simulink model "atrias_HW_boom_nmSt_kinSw"  (R2015a)
settings: Solver=ode4  StartTime=0.0  StopTime=inf  FixedStep=sample_time  RelTol=1e-3
values from neighbouring files (symbols this model uses):
  control_start_time = 15    [setParams.m]
  flag_CtrlMode = 0    [setParams.m]
  kinSw_t_start = 0.5    [setParams.m]
  poser_LLegAlp = (initial_l_leg_angle -pi/2)*180/pi    (= 105)    [setParams.m]
  poser_LLegLen = initial_l_leg_length    (= 0.8)    [setParams.m]
  poser_RLegAlp = (initial_r_leg_angle -pi/2)*180/pi    (= 75)    [setParams.m]
  poser_RLegLen = initial_r_leg_length    (= 0.8)    [setParams.m]
  tune_kinSw_alpha_start = kinSw_alpha_start*180/pi    (= 130)    [setParams.m]
  tune_kinSw_alpha_tgt = kinSw_alpha_tgt*180/pi    (= 80)    [setParams.m]
  tune_kinSw_len_min = kinSw_len_min    (= 0.7)    [setParams.m]
  tune_kinSw_len_tgt = kinSw_len_tgt    (= 0.9)    [setParams.m]
  tune_kinSw_min_t_del = kinSw_min_t_del    (= 0.425)    [setParams.m]
  tune_kinSw_t_del = kinSw_t_del    (= 0.5)    [setParams.m]
  tune_M1_G = St_FGain_VAS*FmaxVAS    [setParams.m]
  tune_M3_0 = CtrlPar_theta0*180/pi    [setParams.m]
  tune_M3_D = St_GainDTh_HFL    [setParams.m]
  tune_M3_P = St_GainTh_HFL    [setParams.m]
undefined symbols (not defined in the file or in its folder): A1_notch_f1, A2_notch_f1, A_kalman_fourbar_gear, A_lpf_dtau, B1_lpf_dtau, B1_notch_f1, B2_lpf_dtau, B2_notch_f1, B_kalman_fourbar_gear, boom_mount_angle, boom_mount_to_center_diagonal, c_jointstop, C_kalman_fourbar_gear, contactThr, d_vertical_com, delta_phi_max, delta_phi_max_buffer, delta_phi_max_dropoff, delta_phi_min, Discrete, FmaxBFSH, FmaxGLU, FmaxHAM, FmaxHFL, FmaxRF, FmaxVAS, FPCtrlPar, g, gain_nodes_sea_torque, HIP_MTR_MAX_CONT_TORQUE, initial_dx_estimate, j_motor, k_leg_spring, K_notch_f1, k_sea, kalman_load_to_deflect_transmission, kd_lateral, kd_motor, kd_shin_max, kd_shin_min, kd_splay_max, kd_splay_min, kd_thigh_max, kd_thigh_min, kp_lateral, kp_motor, kp_sea_torque, kp_shin_max, kp_shin_min, kp_splay_max, kp_splay_min, kp_thigh_max, kp_thigh_min, l_boom, l_seg, l_v, lateral_motor_efficiency, lateral_offset, lateral_target_angle_right, lateral_transition_force ... (+124)
libraries: simulink_extras x44, simulink x9, ctrlSharedLib x4
(part 2 of 8)

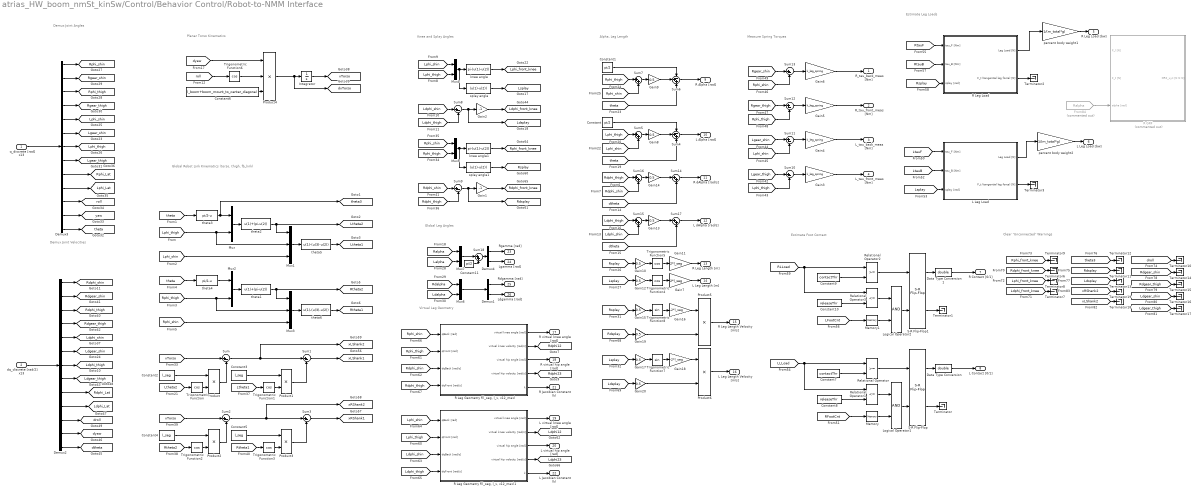
== system atrias_HW_boom_nmSt_kinSw/Control/Behavior Control/Robot-to-NMM Interface ==
  note: Global Robot Link Kinematics
      | (torso, thigh, fb_link)
  note: Planar Torso Kinematics
  note: Alpha, Leg Length
  note: Demux Joint
      | Angles
  note: Demux Joint
      | Velocities
  note: Knee and Splay Angles
  note: Virtual Leg Geometry
  note: Measure Spring Torques
  note: Estimate Leg Loads
  note: Estimate Foot Contact
  note: Clear "Unconnected" Warnings
  note: Global Leg Angles
  q_discrete [rad] x13 : Inport
  dq_discrete [rad/2] x13 : Inport  Port=2
  Constant : Constant  Value=pi/2
  Constant1 : Constant  Value=pi/2
  Constant10 : Constant  Value=releaseThr
  Constant11 : Constant  Value=pi/2
  Constant{2..5} (4 alike) : Constant  Value=l_seg
  Constant6 : Constant  Value=l_boom+boom_mount_to_center_diagonal
  Constant7 : Constant  Value=contactThr
  Constant8 : Constant  Value=releaseThr
  Constant9 : Constant  Value=contactThr
  Data Type Conversion : DataTypeConversion  OutDataTypeStr=double
  Data Type Conversion1 : DataTypeConversion  OutDataTypeStr=double
  Demux1 : Demux  Outputs=2
  Demux2 : Demux  Outputs=13
  Demux3 : Demux  Outputs=13
  Demux4 : Demux  Outputs=2
  From84 : From  Commented=on  GotoTag=Ralpha  TagVisibility=global
  Gain1 : Gain  Gain=-1
  Gain{8..10,12..15,17,19..20} (10 alike) : Gain  Gain=0.5
  Gain11 : Gain  Gain=2*l_seg
  Gain16 : Gain  Gain=-2*l_seg
  Gain18 : Gain  Gain=-2*l_seg
  Gain2 : Gain  Gain=-1
  Gain{3..6} (4 alike) : Gain  Gain=k_leg_spring
  Gain7 : Gain  Gain=2*l_seg
  Integrator : Integrator
  L Leg Load : Subsystem
  Logical Operator1 : Logic  AllPortsSameDT=off  OutDataTypeStr=boolean
  Logical Operator2 : Logic  AllPortsSameDT=off  OutDataTypeStr=boolean
  Memory : Memory
  Memory1 : Memory
  Mux{,2,4..7} (6 alike) : Mux  Inputs=2
  Mux1 : Mux  Inputs=3
  Mux3 : Mux  Inputs=3
  Product{,1..3,5..6} (6 alike) : Product
  Product4 : Product  Inputs=3
  R GRF : Subsystem  Commented=on
  "R Leg Geometry f(l_seg, l_v, v12_max)" : Subsystem
  "R Leg Geometry f(l_seg, l_v, v12_max)1" : Subsystem
  R Leg Load : Subsystem
  Relational Operator : RelationalOperator  OutDataTypeStr=boolean
  Relational Operator1 : RelationalOperator  Operator=<=  OutDataTypeStr=boolean
  Relational Operator2 : RelationalOperator  OutDataTypeStr=boolean
  Relational Operator3 : RelationalOperator  Operator=<=  OutDataTypeStr=boolean
  S-R Flip-Flop : simulink_extras/Flip Flops/S-R Flip-Flop  initial_condition=0
  S-R Flip-Flop1 : simulink_extras/Flip Flops/S-R Flip-Flop  initial_condition=0
  Sum{,1..3,8..13} (10 alike) : Sum  Inputs=|+-
  Sum{5,7,14..18} (7 alike) : Sum  Inputs=|++
  Sum4 : Sum  Inputs=-++
  Sum6 : Sum  Inputs=-++
  Terminator{,1..3,6..19} (18 alike) : Terminator
  Trigonometric Function{,1..6} (7 alike) : Trigonometry  Operator=cos
  Trigonometric Function7 : Trigonometry
  Trigonometric Function8 : Trigonometry
  knee angle : Fcn  Expr=pi-(u(1)-u(2))
  knee angle1 : Fcn  Expr=pi-(u(1)-u(2))
  percent body weight1 : Gain  Gain=1/(m_total*g)
  percent body weight2 : Gain  Gain=1/(m_total*g)
  splay angle : Fcn  Expr=(u(1)-u(2))
  splay angle1 : Fcn  Expr=(u(1)-u(2))
  theta1 : Fcn  Expr=u(1)+(pi-u(2))
  theta2 : Fcn  Expr=u(1)+(pi-u(2))
  theta3 : Fcn  Expr=pi/2-u
  theta4 : Fcn  Expr=pi/2-u
  theta5 : Fcn  Expr=u(1)-(u(3)-u(2))
  theta6 : Fcn  Expr=u(1)-(u(3)-u(2))
  R_tau_back_meas [Nm] : Outport
  R_tau_front_meas [Nm] : Outport  Port=2
  L_tau_back_meas [Nm] : Outport  Port=3
  L_tau_front_meas [Nm] : Outport  Port=4
  R Leg Load [bw] : Outport  Port=5
  L Leg Load [bw] : Outport  Port=6
  R Contact [0/1] : Outport  Port=7
  L Contact [0/1] : Outport  Port=8
  R Alpha [rad] : Outport  Port=9
  L Alpha [rad] : Outport  Port=10
  R dAlpha [rad/s] : Outport  Port=11
  L dAlpha [rad/s] : Outport  Port=12
  R Leg Length [m] : Outport  Port=13
  L Leg Length [m] : Outport  Port=14
  R Leg Length Velocity [m/s] : Outport  Port=15
  L Leg Length Velocity [m/s] : Outport  Port=16
  R virtual knee angle [rad] : Outport  Port=17
  R virtual hip angle [rad] : Outport  Port=18
  L virtual knee angle [rad] : Outport  Port=19
  L virtual hip angle [rad] : Outport  Port=20
  R Jacobian Constant (k) : Outport  Port=21
  L Jacobian Constant (k) : Outport  Port=22
  Rgamma [rad] : Outport  Port=23
  Lgamma [rad] : Outport  Port=24
  Rdgamma [rad] : Outport  Port=25
  Ldgamma [rad] : Outport  Port=26
  tag scope: Ldgear_shin=global, Ldgear_thigh=global, Ldphi12=global, Ldphi23=global, Ldphi_Lat=global, Ldphi_front_knee=global, Ldphi_shin=global, Ldphi_thigh=global, Ldsplay=global, Lgear_shin=global, Lgear_thigh=global, Lphi_Lat=global, Lphi_front_knee=global, Lphi_shin=global, Lphi_thigh=global, Lsplay=global, Ltheta1=global, Ltheta2=global, Rdgear_shin=global, Rdgear_thigh=global, Rdphi12=global, Rdphi23=global, Rdphi_Lat=global, Rdphi_front_knee=global, Rdphi_shin=global, Rdphi_thigh=global, Rdsplay=global, Rgear_shin=global, Rgear_thigh=global, Rphi_Lat=global, Rphi_front_knee=global, Rphi_shin=global, Rphi_thigh=global, Rsplay=global, Rtheta1=global, Rtheta2=global, droll=global, dtheta=global, dxTorso=global, dyaw=global, roll=global, theta3=global, theta=global, xLShank1=global, xLShank2=global, xRShank1=global, xRShank2=global, xTorso=global, yaw=global
  wires:
  Sum3/1 -> [xRShank1]
  Sum2/1 -> [xRShank2], Sum3/1
  Product3/1 -> Sum3/2
  Trigonometric Function3/1 -> Product3/2
  Constant2/1 -> Product/1
  Trigonometric Function/1 -> Product/2
  Sum1/1 -> [xLShank1]
  Constant3/1 -> Product1/1
  Trigonometric Function2/1 -> Product2/2
  Product1/1 -> Sum1/2
  [Rtheta2] -> Trigonometric Function2/1
  Sum/1 -> [xLShank2], Sum1/1
  [Ltheta1] -> Trigonometric Function1/1
  Product/1 -> Sum/2
  Product2/1 -> Sum2/2
  [xTorso] -> Sum2/1
  [Rtheta1] -> Trigonometric Function3/1
  Constant4/1 -> Product2/1
  Constant5/1 -> Product3/1
  [xTorso] -> Sum/1
  [Ltheta2] -> Trigonometric Function/1
  Product4/1 -> [dxTorso], Integrator/1
  Trigonometric Function1/1 -> Product1/2
  Integrator/1 -> [xTorso]
  [dyaw] -> Product4/1
  [theta] -> theta3/1
  [Lphi_thigh] -> Mux1/2, Mux/2
  theta3/1 -> Mux/1, [theta3]
  Mux/1 -> theta2/1
  theta2/1 -> Mux1/1, [Ltheta2]
  Mux1/1 -> theta5/1
  [Lphi_shin] -> Mux1/3
  [theta] -> theta4/1
  [Rphi_thigh] -> Mux3/2, Mux2/2
  theta4/1 -> Mux2/1
  Mux2/1 -> theta1/1
  theta1/1 -> Mux3/1, [Rtheta2]
  Mux3/1 -> theta6/1
  [Rphi_shin] -> Mux3/3
  theta5/1 -> [Ltheta1]
  theta6/1 -> [Rtheta1]
  [theta] -> Sum4/3
  Constant/1 -> Sum4/1
  [Lphi_thigh] -> Sum5/1
  [Lphi_shin] -> Sum5/2
  Sum5/1 -> Gain8/1
  Gain8/1 -> Sum4/2
  Sum4/1 -> L Alpha [rad]/1
  [theta] -> Sum6/3
  Constant1/1 -> Sum6/1
  [Rphi_thigh] -> Sum7/1
  [Rphi_shin] -> Sum7/2
  Sum7/1 -> Gain9/1
  Gain9/1 -> Sum6/2
  Sum6/1 -> R Alpha [rad]/1
  Gain12/1 -> Trigonometric Function4/1
  Gain10/1 -> Trigonometric Function5/1
  Trigonometric Function4/1 -> Gain7/1
  Trigonometric Function5/1 -> Gain11/1
  Demux3/1 -> [Rphi_shin]
  Demux3/2 -> [Rgear_shin]
  Demux3/3 -> [Rphi_thigh]
  Demux3/4 -> [Rgear_thigh]
  Demux3/5 -> [Lphi_shin]
  Demux3/6 -> [Lgear_shin]
  Demux3/7 -> [Lphi_thigh]
  Demux3/8 -> [Lgear_thigh]
  Demux3/9 -> [Rphi_Lat]
  Demux3/10 -> [Lphi_Lat]
  Demux3/11 -> [roll]
  Demux3/12 -> [yaw]
  Demux3/13 -> [theta]
  Demux2/13 -> [dtheta]
  Demux2/8 -> [Ldgear_thigh]
  Demux2/10 -> [Ldphi_Lat]
  Demux2/6 -> [Ldgear_shin]
  Demux2/9 -> [Rdphi_Lat]
  Demux2/11 -> [droll]
  Demux2/12 -> [dyaw]
  Demux2/4 -> [Rdgear_thigh]
  Demux2/5 -> [Ldphi_shin]
  Demux2/7 -> [Ldphi_thigh]
  Demux2/1 -> [Rdphi_shin]
  Demux2/3 -> [Rdphi_thigh]
  Demux2/2 -> [Rdgear_shin]
  q_discrete [rad] x13/1 -> Demux3/1
  dq_discrete [rad/2] x13/1 -> Demux2/1
  Mux4/1 -> splay angle/1, knee angle/1
  [Lphi_thigh] -> Mux4/2
  [Lphi_shin] -> Mux4/1
  knee angle/1 -> [Lphi_front_knee]
  [Ldphi_thigh] -> Sum8/2
  [Ldphi_shin] -> Sum8/1
  Sum8/1 -> [Ldsplay], Gain2/1
  Gain2/1 -> [Ldphi_front_knee]
  splay angle/1 -> [Lsplay]
  Trigonometric Function6/1 -> Product4/2
  [roll] -> Trigonometric Function6/1
  Constant6/1 -> Product4/3
  Mux5/1 -> splay angle1/1, knee angle1/1
  [Rphi_thigh] -> Mux5/2
  [Rphi_shin] -> Mux5/1
  knee angle1/1 -> [Rphi_front_knee]
  [Rdphi_thigh] -> Sum9/2
  [Rdphi_shin] -> Sum9/1
  Sum9/1 -> [Rdsplay], Gain1/1
  Gain1/1 -> [Rdphi_front_knee]
  splay angle1/1 -> [Rsplay]
  [Lgear_shin] -> Sum11/1
  Sum11/1 -> Gain4/1
  [Lphi_shin] -> Sum11/2
  Gain4/1 -> L_tau_back_meas [Nm]/1
  [Lgear_thigh] -> Sum10/1
  Sum10/1 -> Gain3/1
  [Lphi_thigh] -> Sum10/2
  Gain3/1 -> L_tau_front_meas [Nm]/1
  [Rgear_shin] -> Sum13/1
  Sum13/1 -> Gain6/1
  [Rphi_shin] -> Sum13/2
  Gain6/1 -> R_tau_back_meas [Nm]/1
  [Rgear_thigh] -> Sum12/1
  Sum12/1 -> Gain5/1
  [Rphi_thigh] -> Sum12/2
  Gain5/1 -> R_tau_front_meas [Nm]/1
  [Lsplay] -> L Leg Load/3(splay [rad])
  L Leg Load/1(Leg Load [N]) -> percent body weight2/1
  [LtauF] -> L Leg Load/1(tau_F [Nm])
  [LtauB] -> L Leg Load/2(tau_B [Nm])
  percent body weight2/1 -> L Leg Load [bw]/1
  Relational Operator/1 -> S-R Flip-Flop/1
  Constant7/1 -> Relational Operator/2
  S-R Flip-Flop/2 -> Terminator/1
  Logical Operator1/1 -> S-R Flip-Flop/2
  [RFootCnt] -> Memory/1
  Constant8/1 -> Relational Operator1/2
  Relational Operator1/1 -> Logical Operator1/1
  Memory/1 -> Logical Operator1/2
  Data Type Conversion/1 -> L Contact [0/1]/1
  S-R Flip-Flop/1 -> Data Type Conversion/1
  [LLLoad] -> Relational Operator/1, Relational Operator1/1
  [Rsplay] -> R Leg Load/3(splay [rad])
  R Leg Load/1(Leg Load [N]) -> percent body weight1/1
  [RtauF] -> R Leg Load/1(tau_F [Nm])
  [RtauB] -> R Leg Load/2(tau_B [Nm])
  percent body weight1/1 -> R Leg Load [bw]/1
  Relational Operator2/1 -> S-R Flip-Flop1/1
  Constant9/1 -> Relational Operator2/2
  S-R Flip-Flop1/2 -> Terminator1/1
  Logical Operator2/1 -> S-R Flip-Flop1/2
  [LFootCnt] -> Memory1/1
  Constant10/1 -> Relational Operator3/2
  Relational Operator3/1 -> Logical Operator2/1
  Memory1/1 -> Logical Operator2/2
  Data Type Conversion1/1 -> R Contact [0/1]/1
  S-R Flip-Flop1/1 -> Data Type Conversion1/1
  [RLLoad] -> Relational Operator3/1, Relational Operator2/1
  [Rsplay] -> Gain10/1
  [Lsplay] -> Gain12/1
  Gain11/1 -> R Leg Length [m]/1
  Gain7/1 -> L Leg Length [m]/1
  [Rphi_thigh] -> "R Leg Geometry f(l_seg, l_v, v12_max)"/2(qFront [rad])
  [Rphi_shin] -> "R Leg Geometry f(l_seg, l_v, v12_max)"/1(qBack [rad])
  [Rdphi_shin] -> "R Leg Geometry f(l_seg, l_v, v12_max)"/3(dqBack [rad/s])
  [Rdphi_thigh] -> "R Leg Geometry f(l_seg, l_v, v12_max)"/4(dqFront [rad/s])
  "R Leg Geometry f(l_seg, l_v, v12_max)"/4(virtual hip velocity [rad/s]) -> [Rdphi23]
  "R Leg Geometry f(l_seg, l_v, v12_max)"/2(virtual knee velocity [rad/s]) -> [Rdphi12]
  "R Leg Geometry f(l_seg, l_v, v12_max)"/5(k) -> R Jacobian Constant (k)/1
  [Lphi_thigh] -> "R Leg Geometry f(l_seg, l_v, v12_max)1"/2(qFront [rad])
  [Lphi_shin] -> "R Leg Geometry f(l_seg, l_v, v12_max)1"/1(qBack [rad])
  [Ldphi_shin] -> "R Leg Geometry f(l_seg, l_v, v12_max)1"/3(dqBack [rad/s])
  [Ldphi_thigh] -> "R Leg Geometry f(l_seg, l_v, v12_max)1"/4(dqFront [rad/s])
  "R Leg Geometry f(l_seg, l_v, v12_max)1"/5(k) -> L Jacobian Constant (k)/1
  "R Leg Geometry f(l_seg, l_v, v12_max)"/3(virtual hip angle [rad]) -> R virtual hip angle [rad]/1
  "R Leg Geometry f(l_seg, l_v, v12_max)"/1(virtual knee angle [rad]) -> R virtual knee angle [rad]/1
  "R Leg Geometry f(l_seg, l_v, v12_max)1"/1(virtual knee angle [rad]) -> L virtual knee angle [rad]/1
  "R Leg Geometry f(l_seg, l_v, v12_max)1"/3(virtual hip angle [rad]) -> L virtual hip angle [rad]/1
  "R Leg Geometry f(l_seg, l_v, v12_max)1"/2(virtual knee velocity [rad/s]) -> [Ldphi12]
  "R Leg Geometry f(l_seg, l_v, v12_max)1"/4(virtual hip velocity [rad/s]) -> [Ldphi23]
  [Rdphi_front_knee] -> Terminator6/1
  [Ldphi_front_knee] -> Terminator7/1
  [Lphi_front_knee] -> Terminator8/1
  [Rphi_front_knee] -> Terminator9/1
  [droll] -> Terminator10/1
  [Rdsplay] -> Terminator11/1
  [theta3] -> Terminator12/1
  [Ldsplay] -> Terminator13/1
  [Rdgear_shin] -> Terminator14/1
  [Rdgear_thigh] -> Terminator15/1
  [Ldgear_shin] -> Terminator16/1
  [Ldgear_thigh] -> Terminator17/1
  [xLShank2] -> Terminator18/1
  [xRShank2] -> Terminator19/1
  Sum17/1 -> L dAlpha [rad/s]/1
  Sum14/1 -> R dAlpha [rad/s]/1
  [Ldphi_thigh] -> Sum15/1
  [Ldphi_shin] -> Sum15/2
  Sum15/1 -> Gain13/1
  Gain13/1 -> Sum17/1
  [dtheta] -> Sum17/2
  [Rdphi_thigh] -> Sum16/1
  [Rdphi_shin] -> Sum16/2
  Sum16/1 -> Gain14/1
  Gain14/1 -> Sum14/1
  [dtheta] -> Sum14/2
  Constant11/1 -> Sum18/2
  [Ralpha] -> Mux7/1
  [Lalpha] -> Mux7/2
  Mux7/1 -> Sum18/1
  Sum18/1 -> Demux4/1
  Demux4/1 -> Rgamma [rad]/1
  Demux4/2 -> Lgamma [rad]/1
  [Rdalpha] -> Mux6/1
  [Ldalpha] -> Mux6/2
  Mux6/1 -> Demux1/1
  Demux1/1 -> Rdgamma [rad]/1
  Demux1/2 -> Ldgamma [rad]/1
  Gain15/1 -> Trigonometric Function8/1
  Trigonometric Function8/1 -> Gain16/1
  [Rsplay] -> Gain15/1
  Gain16/1 -> Product5/1
  [Rdsplay] -> Gain19/1
  Gain19/1 -> Product5/2
  Product5/1 -> R Leg Length Velocity [m/s]/1
  Gain17/1 -> Trigonometric Function7/1
  Trigonometric Function7/1 -> Gain18/1
  [Lsplay] -> Gain17/1
  Gain18/1 -> Product6/1
  [Ldsplay] -> Gain20/1
  Gain20/1 -> Product6/2
  Product6/1 -> L Leg Length Velocity [m/s]/1
  From84/1 -> R GRF/3(alpha [rad])
  R Leg Load/2(F_t (tangential leg force) [N]) -> Terminator2/1
  L Leg Load/2(F_t (tangential leg force) [N]) -> Terminator3/1

== system atrias_HW_boom_nmSt_kinSw/Control/Behavior Control/Subsystem ==
  R legL : Inport
  R phi : Inport  Port=2
  L legL : Inport  Port=3
  L phi : Inport  Port=4
  R BackGear : Inport  Port=5
  R Front Gear : Inport  Port=6
  L BackGear : Inport  Port=7
  L Front Gear : Inport  Port=8
  Lateral Torque Command [Nm Nm] : Inport  Port=9
  Avoid Hitting Mechanical Limits : MATLAB Function  TreatAsAtomicUnit=on
  Avoid Hitting Mechanical Limits1 : MATLAB Function  TreatAsAtomicUnit=on
  Back/Front Motor PD : Subsystem
  Back/Front Motor PD1 : Subsystem
  Constant1 : Constant
  Constant10 : Constant  Value=max_back_bar_angle
  Constant11 : Constant  Value=min_back_bar_angle
  Constant12 : Constant  Value=min_front_bar_angle
  Constant13 : Constant  Value=[0 0 0 0]  OutDataTypeStr=boolean
  Constant2 : Constant  Value=0
  Constant3 : Constant  Value=max_back_bar_angle
  Constant4 : Constant  Value=min_back_bar_angle
  Constant5 : Constant  Value=min_front_bar_angle
  Constant6 : Constant  Value=0
  Constant7 : Constant  Value=0
  Constant8 : Constant  Value=max_front_bar_angle
  Constant9 : Constant  Value=max_front_bar_angle
  Demux{1..4} (4 alike) : Demux  Outputs=2
  Mux{1..9,11} (10 alike) : Mux  Inputs=2
  Mux10 : Mux  Inputs=3
  Selector33 : Selector  InputPortWidth=6  Indices=[1 2 4 5]
  Selector8 : Selector  InputPortWidth=6  Indices=[1 2 5 3 4 6]
  Virtual Leg to Four Bar : MATLAB Function  TreatAsAtomicUnit=on
  Virtual Leg to Four Bar1 : MATLAB Function  TreatAsAtomicUnit=on
  dtau_des : Subsystem
  Motor Torque Command [Nm] x6 : Outport
  SEA Torque Velocity Command [Nm] x4 : Outport  Port=2
  Force / Position Control [1/0] x4 : Outport  Port=3
  wires:
  R phi/1 -> Virtual Leg to Four Bar/4(phi)
  Avoid Hitting Mechanical Limits/3(dback_cmd) -> Mux9/1
  Avoid Hitting Mechanical Limits/1(back_cmd) -> Mux5/1
  Mux6/1 -> Back/Front Motor PD/3(Desired Acceleration [rad/s^2] [back front])
  Constant9/1 -> Avoid Hitting Mechanical Limits/8(max_front_bar_angle)
  Constant11/1 -> Avoid Hitting Mechanical Limits/9(min_back_bar_angle)
  Constant1/1 -> Back/Front Motor PD/6(Right/Left Leg [1/0])
  R Front Gear/1 -> Demux1/1
  Constant12/1 -> Avoid Hitting Mechanical Limits/7(min_front_bar_angle)
  Demux1/1 -> Mux8/2
  Demux1/2 -> Mux11/2
  Virtual Leg to Four Bar/1(back) -> Avoid Hitting Mechanical Limits/1(back_desired)
  Virtual Leg to Four Bar/2(dback) -> Avoid Hitting Mechanical Limits/2(dback_desired)
  Demux2/1 -> Mux8/1
  Avoid Hitting Mechanical Limits/2(front_cmd) -> Mux5/2
  Virtual Leg to Four Bar/5(dfront) -> Avoid Hitting Mechanical Limits/5(dfront_desired)
  Demux2/2 -> Mux11/1
  R BackGear/1 -> Demux2/1
  Virtual Leg to Four Bar/4(front) -> Avoid Hitting Mechanical Limits/4(front_desired)
  Back/Front Motor PD/1(Commanded Torque [Nm] [back front]) -> [RCommandTorque_back_front]
  Virtual Leg to Four Bar/6(ddfront) -> Avoid Hitting Mechanical Limits/6(ddfront_desired)
  Mux11/1 -> Back/Front Motor PD/5(Measured Velocity [rad/s] [back front])
  Mux8/1 -> Back/Front Motor PD/4(Measured Position [rad] [back front])
  Mux5/1 -> Back/Front Motor PD/1(Desired Position [rad] [back front])
  Virtual Leg to Four Bar/3(ddback) -> Avoid Hitting Mechanical Limits/3(ddback_desired)
  Constant10/1 -> Avoid Hitting Mechanical Limits/10(max_back_bar_angle)
  R legL/1 -> Virtual Leg to Four Bar/1(l_leg)
  Avoid Hitting Mechanical Limits/6(ddfront_cmd) -> Mux6/2
  Avoid Hitting Mechanical Limits/4(dfront_cmd) -> Mux9/2
  Mux9/1 -> Back/Front Motor PD/2(Desired Velocity [rad/s] [back front])
  Avoid Hitting Mechanical Limits/5(ddback_cmd) -> Mux6/1
  Constant7/1 -> Virtual Leg to Four Bar/3(ddl_leg), Virtual Leg to Four Bar/5(dphi), Virtual Leg to Four Bar/6(ddphi), Virtual Leg to Four Bar/2(dl_leg)
  L phi/1 -> Virtual Leg to Four Bar1/4(phi)
  Avoid Hitting Mechanical Limits1/3(dback_cmd) -> Mux7/1
  Avoid Hitting Mechanical Limits1/1(back_cmd) -> Mux2/1
  Mux3/1 -> Back/Front Motor PD1/3(Desired Acceleration [rad/s^2] [back front])
  Constant8/1 -> Avoid Hitting Mechanical Limits1/8(max_front_bar_angle)
  Constant4/1 -> Avoid Hitting Mechanical Limits1/9(min_back_bar_angle)
  Constant2/1 -> Back/Front Motor PD1/6(Right/Left Leg [1/0])
  L Front Gear/1 -> Demux3/1
  Constant5/1 -> Avoid Hitting Mechanical Limits1/7(min_front_bar_angle)
  Demux3/1 -> Mux4/2
  Demux3/2 -> Mux1/2
  Virtual Leg to Four Bar1/1(back) -> Avoid Hitting Mechanical Limits1/1(back_desired)
  Virtual Leg to Four Bar1/2(dback) -> Avoid Hitting Mechanical Limits1/2(dback_desired)
  Demux4/1 -> Mux4/1
  Avoid Hitting Mechanical Limits1/2(front_cmd) -> Mux2/2
  Virtual Leg to Four Bar1/5(dfront) -> Avoid Hitting Mechanical Limits1/5(dfront_desired)
  Demux4/2 -> Mux1/1
  L BackGear/1 -> Demux4/1
  Virtual Leg to Four Bar1/4(front) -> Avoid Hitting Mechanical Limits1/4(front_desired)
  Back/Front Motor PD1/1(Commanded Torque [Nm] [back front]) -> [LCommandTorque_back_front]
  Virtual Leg to Four Bar1/6(ddfront) -> Avoid Hitting Mechanical Limits1/6(ddfront_desired)
  Mux1/1 -> Back/Front Motor PD1/5(Measured Velocity [rad/s] [back front])
  Mux4/1 -> Back/Front Motor PD1/4(Measured Position [rad] [back front])
  Mux2/1 -> Back/Front Motor PD1/1(Desired Position [rad] [back front])
  Virtual Leg to Four Bar1/3(ddback) -> Avoid Hitting Mechanical Limits1/3(ddback_desired)
  Constant3/1 -> Avoid Hitting Mechanical Limits1/10(max_back_bar_angle)
  L legL/1 -> Virtual Leg to Four Bar1/1(l_leg)
  Avoid Hitting Mechanical Limits1/6(ddfront_cmd) -> Mux3/2
  Avoid Hitting Mechanical Limits1/4(dfront_cmd) -> Mux7/2
  Mux7/1 -> Back/Front Motor PD1/2(Desired Velocity [rad/s] [back front])
  Avoid Hitting Mechanical Limits1/5(ddback_cmd) -> Mux3/1
  Constant6/1 -> Virtual Leg to Four Bar1/3(ddl_leg), Virtual Leg to Four Bar1/5(dphi), Virtual Leg to Four Bar1/6(ddphi), Virtual Leg to Four Bar1/2(dl_leg)
  Constant13/1 -> Force / Position Control [1/0] x4/1
  Lateral Torque Command [Nm Nm]/1 -> Mux10/3
  [LCommandTorque_back_front] -> Mux10/2
  [RCommandTorque_back_front] -> Mux10/1
  Mux10/1 -> Selector8/1
  Selector8/1 -> Selector33/1, Motor Torque Command [Nm] x6/1
  Selector33/1 -> dtau_des/1(x)
  dtau_des/1(dx/dt) -> SEA Torque Velocity Command [Nm] x4/1

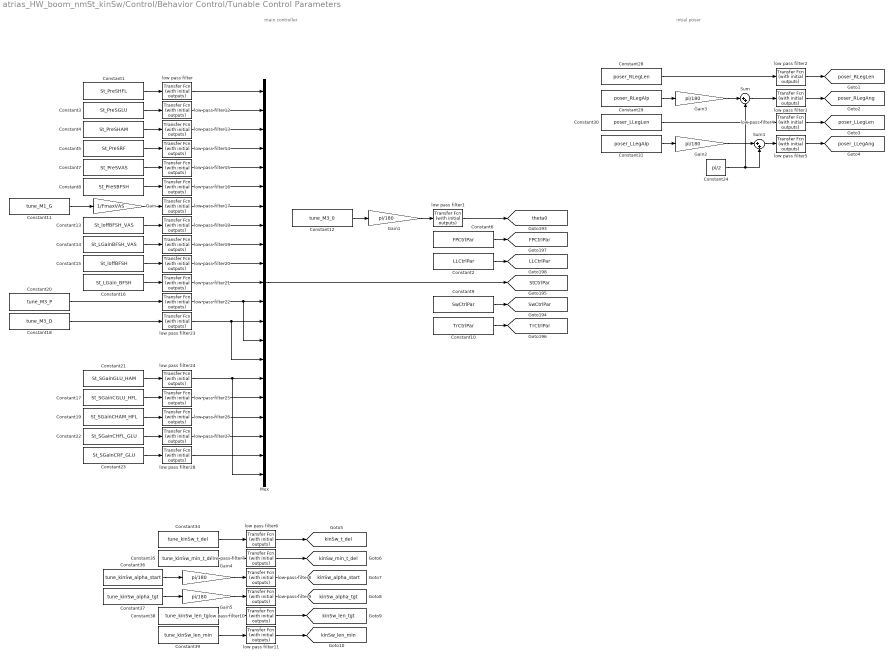
== system atrias_HW_boom_nmSt_kinSw/Control/Behavior Control/Tunable Control Parameters ==
  note: main controller
  note: intial poser
  Constant1 : Constant  Value=St_PreSHFL
  Constant10 : Constant  Value=TrCtrlPar
  Constant11 : Constant  Value=tune_M1_G
  Constant12 : Constant  Value=tune_M3_0
  Constant13 : Constant  Value=St_loffBFSH_VAS
  Constant14 : Constant  Value=St_LGainBFSH_VAS
  Constant15 : Constant  Value=St_loffBFSH
  Constant16 : Constant  Value=St_LGain_BFSH
  Constant17 : Constant  Value=St_SGainCGLU_HFL
  Constant18 : Constant  Value=tune_M3_D
  Constant19 : Constant  Value=St_SGainCHAM_HFL
  Constant2 : Constant  Value=LLCtrlPar
  Constant20 : Constant  Value=tune_M3_P
  Constant21 : Constant  Value=St_SGainGLU_HAM
  Constant22 : Constant  Value=St_SGainCHFL_GLU
  Constant23 : Constant  Value=St_SGainCRF_GLU
  Constant24 : Constant  Value=pi/2
  Constant28 : Constant  Value=poser_RLegLen
  Constant29 : Constant  Value=poser_RLegAlp
  Constant3 : Constant  Value=St_PreSGLU
  Constant30 : Constant  Value=poser_LLegLen
  Constant31 : Constant  Value=poser_LLegAlp
  Constant34 : Constant  Value=tune_kinSw_t_del
  Constant35 : Constant  Value=tune_kinSw_min_t_del
  Constant36 : Constant  Value=tune_kinSw_alpha_start
  Constant37 : Constant  Value=tune_kinSw_alpha_tgt
  Constant38 : Constant  Value=tune_kinSw_len_tgt
  Constant39 : Constant  Value=tune_kinSw_len_min
  Constant4 : Constant  Value=St_PreSHAM
  Constant5 : Constant  Value=St_PreSRF
  Constant6 : Constant  Value=FPCtrlPar
  Constant7 : Constant  Value=St_PreSVAS
  Constant8 : Constant  Value=St_PreSBFSH
  Constant9 : Constant  Value=SwCtrlPar
  Gain : Gain  Gain=1/FmaxVAS
  Gain{1..5} (5 alike) : Gain  Gain=pi/180
  Mux : Mux  Inputs=21
  Sum : Sum  Inputs=|++
  Sum1 : Sum  Inputs=|++
  low pass filter{,1..28} (29 alike) : simulink_extras/Additional Linear/Transfer Fcn (with initial outputs)  N=[1]  D="[.5  1]"  Y0=0  U0=0
      settings: AttributesFormatString=pre-activation: %<Y0>
  tag scope: FPCtrlPar=global, LLCtrlPar=global, StCtrlPar=global, SwCtrlPar=global, TrCtrlPar=global, kinSw_alpha_start=global, kinSw_alpha_tgt=global, kinSw_len_min=global, kinSw_len_tgt=global, kinSw_min_t_del=global, kinSw_t_del=global, poser_LLegAng=global, poser_LLegLen=global, poser_RLegAng=global, poser_RLegLen=global, theta0=global
  wires:
  Constant6/1 -> [FPCtrlPar]
  Constant10/1 -> [TrCtrlPar]
  Constant9/1 -> [SwCtrlPar]
  Constant2/1 -> [LLCtrlPar]
  Constant12/1 -> Gain1/1
  Constant11/1 -> Gain/1
  Mux/1 -> [StCtrlPar]
  low pass filter1/1 -> [theta0]
  Gain1/1 -> low pass filter1/1
  Constant1/1 -> low pass filter/1
  Constant3/1 -> low pass filter12/1
  Constant4/1 -> low pass filter13/1
  Constant5/1 -> low pass filter14/1
  Constant7/1 -> low pass filter15/1
  Constant8/1 -> low pass filter16/1
  Gain/1 -> low pass filter17/1
  Constant13/1 -> low pass filter18/1
  Constant14/1 -> low pass filter19/1
  Constant15/1 -> low pass filter20/1
  Constant16/1 -> low pass filter21/1
  Constant20/1 -> low pass filter22/1
  Constant18/1 -> low pass filter23/1
  Constant21/1 -> low pass filter24/1
  Constant17/1 -> low pass filter25/1
  Constant19/1 -> low pass filter26/1
  Constant22/1 -> low pass filter27/1
  Constant23/1 -> low pass filter28/1
  Constant28/1 -> low pass filter2/1
  Constant30/1 -> low pass filter4/1
  low pass filter2/1 -> [poser_RLegLen]
  low pass filter3/1 -> [poser_RLegAng]
  low pass filter4/1 -> [poser_LLegLen]
  low pass filter5/1 -> [poser_LLegAng]
  Constant34/1 -> low pass filter6/1
  Constant35/1 -> low pass filter7/1
  Constant36/1 -> Gain4/1
  Constant37/1 -> Gain5/1
  Constant38/1 -> low pass filter10/1
  Constant39/1 -> low pass filter11/1
  low pass filter6/1 -> [kinSw_t_del]
  low pass filter7/1 -> [kinSw_min_t_del]
  low pass filter8/1 -> [kinSw_alpha_start]
  low pass filter9/1 -> [kinSw_alpha_tgt]
  low pass filter10/1 -> [kinSw_len_tgt]
  low pass filter11/1 -> [kinSw_len_min]
  Sum/1 -> low pass filter3/1
  Sum1/1 -> low pass filter5/1
  Constant29/1 -> Gain3/1
  Constant31/1 -> Gain2/1
  Gain2/1 -> Sum1/1
  Gain3/1 -> Sum/1
  Constant24/1 -> Sum/2, Sum1/2
  Gain4/1 -> low pass filter8/1
  Gain5/1 -> low pass filter9/1
  low pass filter/1 -> Mux/1
  low pass filter12/1 -> Mux/2
  low pass filter13/1 -> Mux/3
  low pass filter14/1 -> Mux/4
  low pass filter15/1 -> Mux/5
  low pass filter16/1 -> Mux/6
  low pass filter17/1 -> Mux/7
  low pass filter18/1 -> Mux/8
  low pass filter19/1 -> Mux/9
  low pass filter20/1 -> Mux/10
  low pass filter21/1 -> Mux/11
  low pass filter22/1 -> Mux/14, Mux/12
  low pass filter23/1 -> Mux/15, Mux/13
  low pass filter24/1 -> Mux/21, Mux/16
  low pass filter25/1 -> Mux/17
  low pass filter26/1 -> Mux/18
  low pass filter27/1 -> Mux/19
  low pass filter28/1 -> Mux/20

== system atrias_HW_boom_nmSt_kinSw/Control/Behavior Control/Virtual Neuromuscular Control ==
  note: High-Level
      | Control
  note: Neural
      | Control
  note: Muscle
      | Dynamics
  note: Jacobian Mapping
  Higher Control Layer : Subsystem
  Muscle Layer : Subsystem
  Neural Control Layer : Subsystem
  Torque Distribution : Subsystem
  RtauB_des [Nm] : Outport
  RtauF_des [Nm] : Outport  Port=2
  LtauB_des [Nm] : Outport  Port=3
  LtauF_des [Nm] : Outport  Port=4
  tag scope: Jinv_trans_L=global, Jinv_trans_R=global
  wires:
  Torque Distribution/6(L J_inv_transpose [2x2]) -> [Jinv_trans_L]
  Torque Distribution/5(L tauF [Nm]) -> LtauF_des [Nm]/1
  Torque Distribution/4(L tauB [Nm]) -> LtauB_des [Nm]/1
  Torque Distribution/3(R J_inv_transpose [2x2]) -> [Jinv_trans_R]
  [LM12] -> Torque Distribution/4(L tauK_des [Nm])  "Lknee"
  [LM23] -> Torque Distribution/5(L tauH_des [Nm])  "Lhip"
  [k_R] -> Torque Distribution/3(R Jacobian Constant (k))
  [k_L] -> Torque Distribution/6(L Jacobian Constant (k))
  Torque Distribution/1(R tauB [Nm]) -> RtauB_des [Nm]/1
  Torque Distribution/2(R tauF [Nm]) -> RtauF_des [Nm]/1
  [RM23] -> Torque Distribution/2(R tauH_des [Nm])  "Rhip"
  [RM12] -> Torque Distribution/1(R tauK_des [Nm])  "Rknee"

== system atrias_HW_boom_nmSt_kinSw/Control/Behavior Control/command routing ==
  nm_command : Inport
  kinSw_command : Inport  Port=2
  inSwing [1/0] : Inport  Port=3
  SwLeg (right/left) [1/0] : Inport  Port=4
  Desired Torque Derivative (left) : Subsystem
  Desired Torque Derivative (right) : Subsystem
  Logical Operator : Logic  AllPortsSameDT=off  OutDataTypeStr=boolean
  Logical Operator1 : Logic  Operator=NOT  AllPortsSameDT=off  OutDataTypeStr=boolean
  Logical Operator2 : Logic  AllPortsSameDT=off  OutDataTypeStr=boolean
  Logical Operator3 : Logic  Operator=NOT  AllPortsSameDT=off
  Logical Operator4 : Logic  Operator=NOT  AllPortsSameDT=off
  Mux2 : Mux  Inputs=3
  Mux4 : Mux  Inputs=2
  Mux6 : Mux
  Selector1 : Selector  InputPortWidth=6  Indices=[1 2]
  Selector2 : Selector  InputPortWidth=6  Indices=[3 6]
  Selector3 : Selector  InputPortWidth=6  Indices=[4 5]
  Selector33 : Selector  InputPortWidth=6  Indices=[1 2]
  Selector4 : Selector  InputPortWidth=6  Indices=[4 5]
  Selector5 : Selector  InputPortWidth=6  Indices=[1 2 5 3 4 6]
  Switch1 : Switch  Threshold=0.5
  Switch2 : Switch  Threshold=0.5
  Motor Torque Command [Nm] x6 : Outport
  SEA Torque Velocity Command [Nm] x4 : Outport  Port=2
  Force / Position Control [1/0] x4 : Outport  Port=3
  wires:
  Logical Operator2/1 -> Switch2/2, Logical Operator4/1, Desired Torque Derivative (left)/2(flight [1/0])  "LLeg in Swing"
  nm_command/1 -> Selector3/1, Selector2/1, Selector1/1
  Selector33/1 -> Desired Torque Derivative (right)/1(x)
  inSwing [1/0]/1 -> Logical Operator2/1, Logical Operator/1
  Logical Operator1/1 -> Logical Operator2/2
  Selector3/1 -> Switch2/3
  SwLeg (right/left) [1/0]/1 -> Logical Operator1/1, Logical Operator/2
  Logical Operator/1 -> Logical Operator3/1, Desired Torque Derivative (right)/2(flight [1/0]), Switch1/2  "RLeg in Swing"
  Selector2/1 -> Mux2/3
  Selector1/1 -> Switch1/3
  kinSw_command/1 -> Switch2/1, Switch1/1
  Switch1/1 -> Mux2/1
  Switch2/1 -> Mux2/2
  Mux4/1 -> SEA Torque Velocity Command [Nm] x4/1
  Desired Torque Derivative (left)/1(dx/dt) -> Mux4/2
  Selector4/1 -> Desired Torque Derivative (left)/1(x)
  Desired Torque Derivative (right)/1(dx/dt) -> Mux4/1
  Mux6/1 -> Force / Position Control [1/0] x4/1
  Mux2/1 -> Selector5/1
  Selector5/1 -> Motor Torque Command [Nm] x6/1, Selector33/1, Selector4/1
  Logical Operator3/1 -> Mux6/2, Mux6/1
  Logical Operator4/1 -> Mux6/4, Mux6/3

== system atrias_HW_boom_nmSt_kinSw/Control/Behavior Control/kinematic swing leg controller ==
  note: Convert Leg Angle + Leg Length
      | to Fourbar Angles
  note: PD Control Fourbar Motors
  note: Create Parabolic
      | Trajectory for Leg Angle and Leg Length
  note: Leg Selection
  Ctrl On [1/0] : Inport
  Rstance [1/0] : Inport  Port=2
  Lstance [1/0] : Inport  Port=3
  Ralpha [rad] : Inport  Port=4
  Lalpha [rad] : Inport  Port=5
  Rlength [m] : Inport  Port=6
  Llength [m] : Inport  Port=7
  Rdalpha [rad/s] : Inport  Port=8
  Ldalpha [rad/s] : Inport  Port=9
  theta [rad] : Inport  Port=10
  RBack Gear [rad rad/s] : Inport  Port=11
  RFront Gear [rad rad/s] : Inport  Port=12
  LBack Gear [rad rad/s] : Inport  Port=13
  LFront Gear [rad rad/s] : Inport  Port=14
  t_del [sec] : Inport  Port=15
  min_t_del [sec] : Inport  Port=16
  alpha_init : Inport  Port=17
  alpha_tgt [m] : Inport  Port=18
  Llen_tgt [m] : Inport  Port=19
  lclr_tgt [m] : Inport  Port=20
  Avoid Hitting Mechanical Limits : MATLAB Function  TreatAsAtomicUnit=on
  Back/Front Motor PD : Subsystem
  Clock : Clock
  Constant1 : Constant  Value=max_front_bar_angle
  Constant2 : Constant  Value=max_back_bar_angle
  Constant3 : Constant  Value=min_back_bar_angle
  Constant4 : Constant  Value=pi/2
  Constant7 : Constant  Value=min_front_bar_angle
  Demux : Demux
  Demux1 : Demux  Outputs=2
  Demux2 : Demux  Outputs=3
  Demux3 : Demux  Outputs=2
  Demux4 : Demux  Outputs=3
  Enabled Subsystem : Subsystem  TreatAsAtomicUnit=on
  Enabled Subsystem1 : Subsystem  TreatAsAtomicUnit=on
  Gain1 : Gain  Gain=180/pi
  Gain2 : Gain  Gain=180/pi
  Generate Parabolic Leg Trajectories : MATLAB Function  TreatAsAtomicUnit=on
  Mux : Mux
  Mux{1..5,11} (6 alike) : Mux  Inputs=2
  Mux6 : Mux  Inputs=3
  Sum : Sum  Inputs=+-|
  Sum1 : Sum  Inputs=+-|
  Sum2 : Sum  Inputs=++-
  Virtual Leg to Four Bar : MATLAB Function  TreatAsAtomicUnit=on
  hold : Subsystem
  kinSwCtrl monitor : Scope  NumInputPorts=6
      settings: YMin=-0.1~-0.1~-0.1~80~-400~0.7  YMax=1.1~1.1~1.1~150~300~0.95  SaveName=ScopeData13
  swing leg selector : Subsystem
  Back/Front Motor Torque [Nm Nm] : Outport  InitialOutput=[0 0]
  inSw [1/0] : Outport  Port=2  InitialOutput=0
  SwLeg (right/left) [1/0] : Outport  Port=3  InitialOutput=0
  wires:
  Back/Front Motor PD/1(Commanded Torque [Nm] [back front]) -> Back/Front Motor Torque [Nm Nm]/1
  Rstance [1/0]/1 -> swing leg selector/2(Rstance)
  Lstance [1/0]/1 -> swing leg selector/3(Lstance)
  swing leg selector/1(start swing [1/0]) -> [SwInit]
  swing leg selector/2(swing leg (right/left) [1/0]) -> [RightLeft]
  [SwInit] -> hold/Trigger
  swing leg selector/4(alpha) -> [alpha]
  swing leg selector/5(length) -> [length]
  Virtual Leg to Four Bar/1(back) -> Avoid Hitting Mechanical Limits/1(back_desired)
  Virtual Leg to Four Bar/2(dback) -> Avoid Hitting Mechanical Limits/2(dback_desired)
  Virtual Leg to Four Bar/3(ddback) -> Avoid Hitting Mechanical Limits/3(ddback_desired)
  Virtual Leg to Four Bar/4(front) -> Avoid Hitting Mechanical Limits/4(front_desired)
  Virtual Leg to Four Bar/5(dfront) -> Avoid Hitting Mechanical Limits/5(dfront_desired)
  Virtual Leg to Four Bar/6(ddfront) -> Avoid Hitting Mechanical Limits/6(ddfront_desired)
  Mux11/1 -> Back/Front Motor PD/5(Measured Velocity [rad/s] [back front])
  Mux4/1 -> Back/Front Motor PD/4(Measured Position [rad] [back front])
  Mux1/1 -> Back/Front Motor PD/1(Desired Position [rad] [back front])
  Demux3/2 -> Mux11/1
  Demux3/1 -> Mux4/1
  Avoid Hitting Mechanical Limits/2(front_cmd) -> Mux1/2
  Avoid Hitting Mechanical Limits/1(back_cmd) -> Mux1/1
  [BackGear] -> Demux3/1
  Avoid Hitting Mechanical Limits/3(dback_cmd) -> Mux5/1
  Avoid Hitting Mechanical Limits/4(dfront_cmd) -> Mux5/2
  Avoid Hitting Mechanical Limits/5(ddback_cmd) -> Mux2/1
  Avoid Hitting Mechanical Limits/6(ddfront_cmd) -> Mux2/2
  Mux5/1 -> Back/Front Motor PD/2(Desired Velocity [rad/s] [back front])
  Mux2/1 -> Back/Front Motor PD/3(Desired Acceleration [rad/s^2] [back front])
  [RightLeft] -> Back/Front Motor PD/6(Right/Left Leg [1/0])
  Sum1/1 -> Sum/2
  Sum/1 -> Generate Parabolic Leg Trajectories/3(time_remaining)
  t_del [sec]/1 -> Sum/1, Generate Parabolic Leg Trajectories/2(est_duration)
  swing leg selector/3(flight) -> [flight]
  min_t_del [sec]/1 -> Generate Parabolic Leg Trajectories/10(min_f_duration)
  alpha_tgt [m]/1 -> Mux3/2, Generate Parabolic Leg Trajectories/7(legAlp_star)
  Llen_tgt [m]/1 -> Mux6/2, Generate Parabolic Leg Trajectories/8(legLen_star)
  lclr_tgt [m]/1 -> Mux6/3, Generate Parabolic Leg Trajectories/9(legLen_min)
  Ralpha [rad]/1 -> swing leg selector/4(Ralpha)
  Lalpha [rad]/1 -> swing leg selector/5(Lalpha)
  Rlength [m]/1 -> swing leg selector/6(Rlength)
  Llength [m]/1 -> swing leg selector/7(Llength)
  Rdalpha [rad/s]/1 -> swing leg selector/8(Rdalpha)
  Ldalpha [rad/s]/1 -> swing leg selector/9(Ldalpha)
  swing leg selector/6(dalpha) -> [dalpha]
  Clock/1 -> Sum1/1, Mux/1
  [alpha] -> Mux/2
  [dalpha] -> Mux/3
  [length] -> Mux/4
  Mux/1 -> hold/1(data)
  hold/2(data_SwStart) -> Demux/1
  Demux/1 -> Sum1/2
  Demux/2 -> Generate Parabolic Leg Trajectories/4(legAlp0)
  Demux/3 -> Generate Parabolic Leg Trajectories/5(dlegAlp0)
  Demux/4 -> Generate Parabolic Leg Trajectories/6(legLen0)
  alpha_init/1 -> swing leg selector/14(alpha_init)
  RBack Gear [rad rad/s]/1 -> swing leg selector/10(RBack Gear [rad rad/s])
  RFront Gear [rad rad/s]/1 -> swing leg selector/11(RFront Gear [rad rad/s])
  LBack Gear [rad rad/s]/1 -> swing leg selector/12(LBack Gear [rad rad/s])
  LFront Gear [rad rad/s]/1 -> swing leg selector/13(LFront Gear [rad rad/s])
  swing leg selector/7(Back Gear [rad rad/s]) -> [BackGear]
  swing leg selector/8(Front Gear [rad rad/s]) -> [FrontGear]
  [FrontGear] -> Demux1/1
  Demux1/1 -> Mux4/2
  Demux1/2 -> Mux11/2
  Demux2/1 -> Virtual Leg to Four Bar/1(l_leg)
  Demux2/2 -> Virtual Leg to Four Bar/2(dl_leg)
  Demux2/3 -> Virtual Leg to Four Bar/3(ddl_leg)
  Sum2/1 -> Virtual Leg to Four Bar/4(phi)
  Demux4/2 -> Virtual Leg to Four Bar/5(dphi)
  Demux4/3 -> Virtual Leg to Four Bar/6(ddphi)
  Constant7/1 -> Avoid Hitting Mechanical Limits/7(min_front_bar_angle)
  Constant1/1 -> Avoid Hitting Mechanical Limits/8(max_front_bar_angle)
  Constant3/1 -> Avoid Hitting Mechanical Limits/9(min_back_bar_angle)
  Constant2/1 -> Avoid Hitting Mechanical Limits/10(max_back_bar_angle)
  Demux4/1 -> Sum2/2
  Constant4/1 -> Sum2/1
  Enabled Subsystem/1(Out1) -> Generate Parabolic Leg Trajectories/1(flight)
  [flight] -> Enabled Subsystem/1(In1)
  hold/1(SwCtrlOn) -> [init_SwKinCtrl], Enabled Subsystem/Enable
  Generate Parabolic Leg Trajectories/1(legLen_ref) -> Demux2/1
  Generate Parabolic Leg Trajectories/2(legAlp_ref) -> Demux4/1
  [flight] -> Enabled Subsystem1/1(In1)
  [RightLeft] -> Enabled Subsystem1/2(In2)
  Enabled Subsystem1/2(Out2) -> SwLeg (right/left) [1/0]/1
  Enabled Subsystem1/1(Out1) -> inSw [1/0]/1
  [init_SwKinCtrl] -> Enabled Subsystem1/Enable
  Ctrl On [1/0]/1 -> swing leg selector/1(Ctrl On [1/0])
  [flight] -> kinSwCtrl monitor/3  "flight"
  [SwInit] -> kinSwCtrl monitor/1  "SwInit"
  [RightLeft] -> kinSwCtrl monitor/2  "righ/left"
  [dalpha] -> Gain2/1
  Mux6/1 -> kinSwCtrl monitor/6  "length"
  Gain1/1 -> kinSwCtrl monitor/4  "alpha"
  Gain2/1 -> kinSwCtrl monitor/5  "dalpha"
  [alpha] -> Mux3/1
  Mux3/1 -> Gain1/1
  [length] -> Mux6/1
  theta [rad]/1 -> Sum2/3

== system atrias_HW_boom_nmSt_kinSw/Control/Actuator Control/SEA Controller (Torque)/Antiresonance Compensation ==
  Torque : Inport
  Notch Filter (Flight) : DiscreteTransferFcn  Numerator=[K_notch_f1 K_notch_f1*A1_notch_f1 K_notch_f1*A2_notch_f1]  Denominator=[1 B1_notch_f1 B2_notch_f1]  SampleTime=sample_time
  Filtered Torque : Outport
  wires:
  Notch Filter (Flight)/1 -> Filtered Torque/1
  Torque/1 -> Notch Filter (Flight)/1

== system atrias_HW_boom_nmSt_kinSw/Control/Actuator Control/SEA Controller (Torque)/Friction Compensation ==
  Motor Velocity [rad/s] : Inport
  Gain2 : Gain  Gain=sea_coulomb_friction_direction_switch_sensitivity
  KdGain2 : Gain  Description=xPCTag(1)=kd_sea_torque;  Gain=sea_coulomb_friction
  Trigonometric Function : Trigonometry  Operator=tanh
  Friction Compensation [Nm] : Outport
  wires:
  Trigonometric Function/1 -> KdGain2/1
  Gain2/1 -> Trigonometric Function/1
  Motor Velocity [rad/s]/1 -> Gain2/1
  KdGain2/1 -> Friction Compensation [Nm]/1

== system atrias_HW_boom_nmSt_kinSw/Control/Actuator Control/SEA Controller (Torque)/Loaded Unloaded Switch ==
  Loaded Signal : Inport
  Unloaded Signal : Inport  Port=2
  Loaded/Unloaded [1/0] x4 : Inport  Port=3
  Demux : Demux
  Demux1 : Demux
  Demux2 : Demux
  Mux : Mux
  Switch{,1..3} (4 alike) : Switch  Criteria=u2 ~= 0
  Signal : Outport
  wires:
  Demux2/1 -> Switch/3
  Demux2/2 -> Switch1/3
  Demux2/3 -> Switch2/3
  Demux2/4 -> Switch3/3
  Unloaded Signal/1 -> Demux2/1
  Demux1/4 -> Switch3/1
  Demux1/3 -> Switch2/1
  Demux1/2 -> Switch1/1
  Demux1/1 -> Switch/1
  Loaded Signal/1 -> Demux1/1
  Demux/1 -> Switch/2
  Switch/1 -> Mux/1
  Mux/1 -> Signal/1
  Loaded/Unloaded [1/0] x4/1 -> Demux/1
  Switch3/1 -> Mux/4
  Switch2/1 -> Mux/3
  Switch1/1 -> Mux/2
  Demux/2 -> Switch1/2
  Demux/3 -> Switch2/2
  Demux/4 -> Switch3/2

== system atrias_HW_boom_nmSt_kinSw/Control/Actuator Control/SEA Controller (Torque)/critical damping ==
  p gain : Inport
  Gain : Gain  Gain=1.0
  Gain1 : Gain  Gain=2
  Gain2 : Gain  Gain=j_motor
  Spring Stiffness1 : Gain  Gain=1./k_sea
  Sqrt : Sqrt  SaturateOnIntegerOverflow=on
  d gain : Outport
  wires:
  p gain/1 -> Spring Stiffness1/1
  Gain/1 -> Gain1/1
  Sqrt/1 -> Gain/1
  Gain2/1 -> Sqrt/1
  Spring Stiffness1/1 -> Gain2/1
  Gain1/1 -> d gain/1

== system atrias_HW_boom_nmSt_kinSw/Control/Behavior Control/Add Limit Avoidance PD Torques/mechanical limit avoidance ==
  tau_des [Nm]x4 : Inport
  PD Joint Limit : Subsystem
  Product : Product
  Sum : Sum  Inputs=++|
  tau_des + pd [Nm]x4 : Outport
  wires:
  tau_des [Nm]x4/1 -> Product/2
  PD Joint Limit/1(tau_pd [Nm]x4) -> Sum/1
  Sum/1 -> tau_des + pd [Nm]x4/1
  PD Joint Limit/2(des_trq_scale x4) -> Product/1
  Product/1 -> Sum/2

== system atrias_HW_boom_nmSt_kinSw/Control/Behavior Control/Robot-to-NMM Interface/L Leg Load ==
  tau_F [Nm] : Inport
  tau_B [Nm] : Inport  Port=2
  splay [rad] : Inport  Port=3
  Calculate Leg Load : Fcn  Expr=1/(2*l_seg*sin(u(3)/2))*u(1)-1/(2*l_seg*sin(u(3)/2))*u(2)
  Calculate Tangential Leg Force : Fcn  Expr=1/(2*l_seg*cos(u(3)/2))*(u(1)+u(2))
  Mux : Mux  Inputs=3
  Positive Values only : Saturate  UpperLimit=Inf  LowerLimit=0
  Leg Load [N] : Outport
  F_t (tangential leg force) [N] : Outport  Port=2
  wires:
  Calculate Leg Load/1 -> Positive Values only/1
  Positive Values only/1 -> Leg Load [N]/1
  Mux/1 -> Calculate Tangential Leg Force/1, Calculate Leg Load/1
  splay [rad]/1 -> Mux/3
  tau_B [Nm]/1 -> Mux/2
  tau_F [Nm]/1 -> Mux/1
  Calculate Tangential Leg Force/1 -> F_t (tangential leg force) [N]/1

== system atrias_HW_boom_nmSt_kinSw/Control/Behavior Control/Robot-to-NMM Interface/R GRF ==
  F_l [N] : Inport
  F_t [N] : Inport  Port=2
  alpha [rad] : Inport  Port=3
  Constant : Constant
  GRF tangential (x) : Fcn  Expr=-u(1)*cos(u(3)) + u(2)*sin(u(3))
  GRF vertical : Fcn  Expr=u(1)*sin(u(3)) + u(2)*cos(u(3))
  Mux : Mux  Inputs=3
  Mux1 : Mux  Inputs=3
  GRF_xyz [N N N] : Outport
  wires:
  alpha [rad]/1 -> Mux/3
  F_t [N]/1 -> Mux/2
  F_l [N]/1 -> Mux/1
  Mux/1 -> GRF tangential (x)/1, GRF vertical/1
  GRF tangential (x)/1 -> Mux1/1
  GRF vertical/1 -> Mux1/2

== system atrias_HW_boom_nmSt_kinSw/Control/Behavior Control/Robot-to-NMM Interface/R Leg Geometry f(l_seg, l_v, v12_max) ==
  qBack [rad] : Inport
  qFront [rad] : Inport  Port=2
  dqBack [rad/s] : Inport  Port=3
  dqFront [rad/s] : Inport  Port=4
  Constant : Constant  Value=pi/2
  Constant1 : Constant  Value=l_seg/l_v
  Divide : Product  Inputs=**/
  Fcn : Fcn  Expr=(1-u(3))/2*u(1) + (1+u(3))/2*u(2)
  Fcn1 : Fcn  Expr=-u(3)*u(1) + u(3)*u(2)
  Gain : Gain  Gain=0.5
  Gain1 : Gain  Gain=0.5
  Gain2 : Gain  Gain=l_seg/l_v
  Gain3 : Gain  Gain=2
  Gain4 : Gain  Gain=0.5
  Mux : Mux  Inputs=3
  Sum : Sum  Inputs=|+-
  Sum1 : Sum  Inputs=|+-
  Sum2 : Sum  Inputs=|++
  Sum3 : Sum  Inputs=|++
  Trigonometric Function : Trigonometry  Operator=cos
  Trigonometric Function1 : Trigonometry  Operator=asin
  Trigonometric Function2 : Trigonometry
  Trigonometric Function3 : Trigonometry  Operator=cos
  "[0,sin(v12_max/2)]" : Saturate  UpperLimit=sin(v12_max/2)  LowerLimit=0
  "[0,v12_max]" : Saturate  UpperLimit=v12_max  LowerLimit=0
  "[min_splay_angle/2, inf]" : Saturate  UpperLimit=inf  LowerLimit=min_splay_angle/2
  virtual knee angle [rad] : Outport
  virtual knee velocity [rad/s] : Outport  Port=2
  virtual hip angle [rad] : Outport  Port=3
  virtual hip velocity [rad/s] : Outport  Port=4
  k : Outport  Port=5
  wires:
  Sum/1 -> Gain/1
  qBack [rad]/1 -> [qB]
  qFront [rad]/1 -> [qF]
  dqBack [rad/s]/1 -> [dqB]
  dqFront [rad/s]/1 -> [dqF]
  [qF] -> Sum3/2, Sum/2
  [qB] -> Sum/1, Sum3/1
  Gain/1 -> Trigonometric Function/1, "[min_splay_angle/2, inf]"/1
  [phiK] -> Gain1/1
  Sum1/1 -> Sum2/1
  Constant/1 -> Sum1/2
  Gain1/1 -> Trigonometric Function3/1, Sum2/2
  Sum2/1 -> [phiH]
  Trigonometric Function/1 -> Gain2/1
  Gain2/1 -> "[0,sin(v12_max/2)]"/1
  "[0,sin(v12_max/2)]"/1 -> Trigonometric Function1/1
  Trigonometric Function1/1 -> "[0,v12_max]"/1
  "[0,v12_max]"/1 -> Gain3/1
  Gain3/1 -> [phiK]
  [phiK] -> virtual knee angle [rad]/1
  [phiH] -> virtual hip angle [rad]/1
  Trigonometric Function2/1 -> Divide/2
  Constant1/1 -> Divide/1
  Trigonometric Function3/1 -> Divide/3
  Divide/1 -> k/1, Mux/3
  Mux/1 -> Fcn/1, Fcn1/1
  [dqF] -> Mux/2
  [dqB] -> Mux/1
  Fcn/1 -> virtual hip velocity [rad/s]/1
  Fcn1/1 -> virtual knee velocity [rad/s]/1
  Sum3/1 -> Gain4/1
  Gain4/1 -> Sum1/1
  "[min_splay_angle/2, inf]"/1 -> Trigonometric Function2/1

== system atrias_HW_boom_nmSt_kinSw/Control/Behavior Control/Robot-to-NMM Interface/R Leg Geometry f(l_seg, l_v, v12_max)1 ==
  qBack [rad] : Inport
  qFront [rad] : Inport  Port=2
  dqBack [rad/s] : Inport  Port=3
  dqFront [rad/s] : Inport  Port=4
  Constant : Constant  Value=pi/2
  Constant1 : Constant  Value=l_seg/l_v
  Divide : Product  Inputs=**/
  Fcn : Fcn  Expr=(1-u(3))/2*u(1) + (1+u(3))/2*u(2)
  Fcn1 : Fcn  Expr=-u(3)*u(1) + u(3)*u(2)
  Gain : Gain  Gain=0.5
  Gain1 : Gain  Gain=0.5
  Gain2 : Gain  Gain=l_seg/l_v
  Gain3 : Gain  Gain=2
  Gain4 : Gain  Gain=0.5
  Mux : Mux  Inputs=3
  Sum : Sum  Inputs=|+-
  Sum1 : Sum  Inputs=|+-
  Sum2 : Sum  Inputs=|++
  Sum3 : Sum  Inputs=|++
  Trigonometric Function : Trigonometry  Operator=cos
  Trigonometric Function1 : Trigonometry  Operator=asin
  Trigonometric Function2 : Trigonometry
  Trigonometric Function3 : Trigonometry  Operator=cos
  "[0,sin(v12_max/2)]" : Saturate  UpperLimit=sin(v12_max/2)  LowerLimit=0
  "[0,v12_max]" : Saturate  UpperLimit=v12_max  LowerLimit=0
  "[min_splay_angle/2, inf]" : Saturate  UpperLimit=inf  LowerLimit=min_splay_angle/2
  virtual knee angle [rad] : Outport
  virtual knee velocity [rad/s] : Outport  Port=2
  virtual hip angle [rad] : Outport  Port=3
  virtual hip velocity [rad/s] : Outport  Port=4
  k : Outport  Port=5
  wires:
  "[min_splay_angle/2, inf]"/1 -> Trigonometric Function2/1
  Gain4/1 -> Sum1/1
  Sum3/1 -> Gain4/1
  Fcn1/1 -> virtual knee velocity [rad/s]/1
  Fcn/1 -> virtual hip velocity [rad/s]/1
  [dqB] -> Mux/1
  [dqF] -> Mux/2
  Mux/1 -> Fcn1/1, Fcn/1
  Divide/1 -> Mux/3, k/1
  Trigonometric Function3/1 -> Divide/3
  Constant1/1 -> Divide/1
  Trigonometric Function2/1 -> Divide/2
  [phiH] -> virtual hip angle [rad]/1
  [phiK] -> virtual knee angle [rad]/1
  Gain3/1 -> [phiK]
  "[0,v12_max]"/1 -> Gain3/1
  Trigonometric Function1/1 -> "[0,v12_max]"/1
  "[0,sin(v12_max/2)]"/1 -> Trigonometric Function1/1
  Gain2/1 -> "[0,sin(v12_max/2)]"/1
  Trigonometric Function/1 -> Gain2/1
  Sum2/1 -> [phiH]
  Gain1/1 -> Sum2/2, Trigonometric Function3/1
  Constant/1 -> Sum1/2
  Sum1/1 -> Sum2/1
  [phiK] -> Gain1/1
  Gain/1 -> "[min_splay_angle/2, inf]"/1, Trigonometric Function/1
  [qB] -> Sum3/1, Sum/1
  [qF] -> Sum/2, Sum3/2
  dqFront [rad/s]/1 -> [dqF]
  dqBack [rad/s]/1 -> [dqB]
  qFront [rad]/1 -> [qF]
  qBack [rad]/1 -> [qB]
  Sum/1 -> Gain/1

== system atrias_HW_boom_nmSt_kinSw/Control/Behavior Control/Robot-to-NMM Interface/R Leg Load ==
  tau_F [Nm] : Inport
  tau_B [Nm] : Inport  Port=2
  splay [rad] : Inport  Port=3
  Calculate Leg Load : Fcn  Expr=1/(2*l_seg*sin(u(3)/2))*u(1)-1/(2*l_seg*sin(u(3)/2))*u(2)
  Calculate Tangential Leg Force : Fcn  Expr=1/(2*l_seg*cos(u(3)/2))*(u(1)+u(2))
  Mux : Mux  Inputs=3
  Positive Values only : Saturate  UpperLimit=Inf  LowerLimit=0
  Leg Load [N] : Outport
  F_t (tangential leg force) [N] : Outport  Port=2
  wires:
  Calculate Leg Load/1 -> Positive Values only/1
  Positive Values only/1 -> Leg Load [N]/1
  Mux/1 -> Calculate Tangential Leg Force/1, Calculate Leg Load/1
  splay [rad]/1 -> Mux/3
  tau_B [Nm]/1 -> Mux/2
  tau_F [Nm]/1 -> Mux/1
  Calculate Tangential Leg Force/1 -> F_t (tangential leg force) [N]/1

== system atrias_HW_boom_nmSt_kinSw/Control/Behavior Control/Subsystem/Back//Front Motor PD ==
  Desired Position [rad] [back front] : Inport
  Desired Velocity [rad/s] [back front] : Inport  Port=2
  Desired Acceleration [rad/s^2] [back front] : Inport  Port=3
  Measured Position [rad] [back front] : Inport  Port=4
  Measured Velocity [rad/s] [back front] : Inport  Port=5
  Right/Left Leg [1/0] : Inport  Port=6
  Friction Compensation : Subsystem
  Product : Product
  Sum1 : Sum  Inputs=|++
  Sum2 : Sum  Inputs=|++
  Sum7 : Sum  Inputs=|+-
  Sum8 : Sum  Inputs=|+-
  Sum9 : Sum
  kd : Gain  Gain=kd_motor
  kp : Gain  Gain=kp_motor
  reflected inertia : Constant  Value=j_motor
  Commanded Torque [Nm] [back front] : Outport
  wires:
  kp/1 -> Sum9/1
  Sum7/1 -> kp/1
  Measured Position [rad] [back front]/1 -> Sum7/2
  Sum9/1 -> Sum1/1
  Sum8/1 -> kd/1
  Desired Position [rad] [back front]/1 -> Sum7/1
  kd/1 -> Sum9/2
  Measured Velocity [rad/s] [back front]/1 -> Sum8/2
  Sum1/1 -> Sum2/1
  Desired Acceleration [rad/s^2] [back front]/1 -> Product/1
  Product/1 -> Sum1/2
  Right/Left Leg [1/0]/1 -> Friction Compensation/1(Right/Left [1/0])
  Sum2/1 -> Commanded Torque [Nm] [back front]/1
  Desired Velocity [rad/s] [back front]/1 -> Friction Compensation/2(Commanded Velocity [rad/s] [back front]), Sum8/1
  reflected inertia/1 -> Product/2
  Friction Compensation/1(Friction Compensation [Nm]) -> Sum2/2
